simulink model "cantoni_combined_matrices_6pools_split"  (R2019b)
settings: Solver=FixedStepDiscrete  StartTime=0.0  StopTime=30000  FixedStep=h  RelTol=1e-3
undefined symbols (not defined in the file or in its folder): comb_contr, comb_plant_disc, ddelay, h, Pd, Wd
settings Model: Creator=Jacob  LastModifiedBy=bas
settings SFSimCC: CustomCodeUndefinedFunction=UseInterfaceOnly

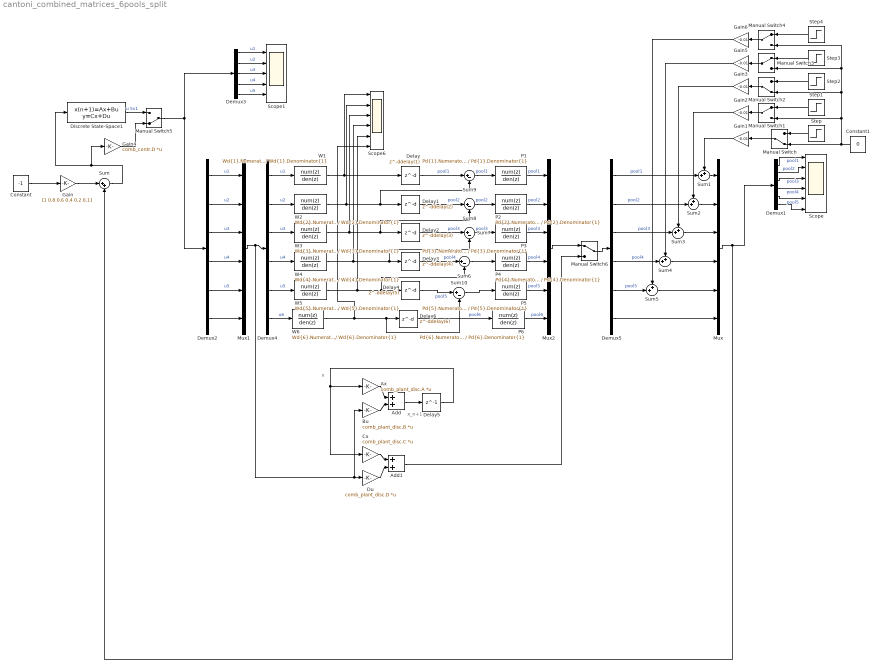
== system cantoni_combined_matrices_6pools_split ==
  note: x
  note: x_n+1
  Add : Sum
  Add1 : Sum
  Ax : Gain  Gain=comb_plant_disc.A  Multiplication=Matrix(K*u)
  Bu : Gain  Gain=comb_plant_disc.B  Multiplication=Matrix(K*u)
  Constant : Constant  Value=-1
  Constant1 : Constant  Value=0
  Cx : Gain  Gain=comb_plant_disc.C  Multiplication=Matrix(K*u)
  Delay : Delay  DelayLength=ddelay(1)
  Delay1 : Delay  DelayLength=ddelay(2)
  Delay2 : Delay  DelayLength=ddelay(3)
  Delay3 : Delay  DelayLength=ddelay(4)
  Delay4 : Delay  DelayLength=ddelay(5)
  Delay5 : Delay  DelayLength=1  InitialCondition=[0;0;0;0;0;0;0;0;0;0;0;0;0;0;0;0;0;0;0;0;0;0;0;0]
  Delay6 : Delay  DelayLength=ddelay(6)
  Demux{1..2,4..5} (4 alike) : Demux  Outputs=6
  Demux3 : Demux  Outputs=5
  Discrete State-Space1 : DiscreteStateSpace  A=comb_contr.A  B=comb_contr.B  C=comb_contr.C  D=comb_contr.D  SampleTime=h
  Du : Gain  Gain=comb_plant_disc.D  Multiplication=Matrix(K*u)
  Gain : Gain  Gain=[1 0.8 0.6 0.4 0.2 0.1]
  Gain{1..3,5..6} (5 alike) : Gain  Gain=-0.01
  Gain4 : Gain  Gain=comb_contr.D  Multiplication=Matrix(K*u)
  Manual Switch : ManualSwitch  CurrentSetting=0
  Manual Switch{1,3..4,6} (4 alike) : ManualSwitch
  Manual Switch2 : ManualSwitch  CurrentSetting=0
  Manual Switch5 : ManualSwitch  CurrentSetting=0
  Mux : Mux  Inputs=6
  Mux1 : Mux  Inputs=6
  Mux2 : Mux  Inputs=6
  P1 : DiscreteTransferFcn  Numerator=Pd{1}.Numerator{1}  Denominator=Pd{1}.Denominator{1}
  P2 : DiscreteTransferFcn  Numerator=Pd{2}.Numerator{1}  Denominator=Pd{2}.Denominator{1}
  P3 : DiscreteTransferFcn  Numerator=Pd{3}.Numerator{1}  Denominator=Pd{3}.Denominator{1}
  P4 : DiscreteTransferFcn  Numerator=Pd{4}.Numerator{1}  Denominator=Pd{4}.Denominator{1}
  P5 : DiscreteTransferFcn  Numerator=Pd{5}.Numerator{1}  Denominator=Pd{5}.Denominator{1}
  P6 : DiscreteTransferFcn  Numerator=Pd{6}.Numerator{1}  Denominator=Pd{6}.Denominator{1}
  Scope : Scope  NumInputPorts=6
  Scope1 : Scope  NumInputPorts=5
  Scope6 : Scope  NumInputPorts=6
  Step{,1..4} (5 alike) : Step  Time=50  SampleTime=0
  Sum : Sum  Inputs=|++
  Sum{1..5} (5 alike) : Sum  Inputs=++|
  Sum{6..10} (5 alike) : Sum  Inputs=|+-
  W1 : DiscreteTransferFcn  Numerator=Wd{1}.Numerator{1}  Denominator=Wd{1}.Denominator{1}
  W2 : DiscreteTransferFcn  Numerator=Wd{2}.Numerator{1}  Denominator=Wd{2}.Denominator{1}
  W3 : DiscreteTransferFcn  Numerator=Wd{3}.Numerator{1}  Denominator=Wd{3}.Denominator{1}
  W4 : DiscreteTransferFcn  Numerator=Wd{4}.Numerator{1}  Denominator=Wd{4}.Denominator{1}
  W5 : DiscreteTransferFcn  Numerator=Wd{5}.Numerator{1}  Denominator=Wd{5}.Denominator{1}
  W6 : DiscreteTransferFcn  Numerator=Wd{6}.Numerator{1}  Denominator=Wd{6}.Denominator{1}
  wires:
  Sum/1 -> Gain4/1, Discrete State-Space1/1
  Constant/1 -> Gain/1
  Gain/1 -> Sum/1
  Mux/1 -> Demux1/1, Sum/2
  Demux1/1 -> Scope/1  "pool1"
  Demux1/2 -> Scope/2  "pool2"
  Demux1/3 -> Scope/3  "pool3"
  Demux1/4 -> Scope/4  "pool4"
  Demux1/5 -> Scope/5  "pool5"
  Step/1 -> Manual Switch/1
  Sum1/1 -> Mux/1
  Demux5/2 -> Sum2/2  "pool2"
  Sum2/1 -> Mux/2
  Gain2/1 -> Sum2/1
  Step1/1 -> Manual Switch1/1
  Gain1/1 -> Sum1/1
  Manual Switch/1 -> Gain1/1
  Constant1/1 -> Manual Switch1/2, Manual Switch4/2, Manual Switch3/2, Manual Switch2/2, Manual Switch/2
  Manual Switch1/1 -> Gain2/1
  Demux5/3 -> Sum3/2  "pool3"
  Sum3/1 -> Mux/3
  Manual Switch2/1 -> Gain3/1
  Step2/1 -> Manual Switch2/1
  Gain3/1 -> Sum3/1
  Demux5/1 -> Sum1/2  "pool1"
  Demux5/4 -> Sum4/2  "pool4"
  Sum4/1 -> Mux/4
  Demux5/5 -> Sum5/2  "pool5"
  Sum5/1 -> Mux/5
  Step3/1 -> Manual Switch3/1
  Manual Switch3/1 -> Gain5/1
  Gain5/1 -> Sum4/1
  Manual Switch4/1 -> Gain6/1
  Step4/1 -> Manual Switch4/1
  Gain6/1 -> Sum5/1
  Demux2/4 -> Mux1/4  "u4"
  Demux2/3 -> Mux1/3  "u3"
  Demux2/2 -> Mux1/2  "u2"
  Demux2/1 -> Mux1/1  "u1"
  Demux2/5 -> Mux1/5  "u5"
  Demux3/5 -> Scope1/5  "u5"
  Demux3/4 -> Scope1/4  "u4"
  Demux3/3 -> Scope1/3  "u3"
  Demux3/2 -> Scope1/2  "u2"
  Demux3/1 -> Scope1/1  "u1"
  W5/1 -> Sum6/2, Delay4/1, Scope6/5
  Discrete State-Space1/1 -> Manual Switch5/1  "u 5x1"
  Manual Switch5/1 -> Demux3/1, Demux2/1
  Gain4/1 -> Manual Switch5/2
  Demux4/1 -> W1/1  "u1"
  Demux4/2 -> W2/1  "u2"
  Demux4/3 -> W3/1  "u3"
  Demux4/4 -> W4/1  "u4"
  Demux4/5 -> W5/1  "u5"
  Mux2/1 -> Manual Switch6/1
  P1/1 -> Mux2/1  "pool1"
  P2/1 -> Mux2/2  "pool2"
  P3/1 -> Mux2/3  "pool3"
  P4/1 -> Mux2/4  "pool4"
  P5/1 -> Mux2/5  "pool5"
  Add1/1 -> Manual Switch6/2
  Manual Switch6/1 -> Demux5/1
  Sum6/1 -> P4/1
  W4/1 -> Sum7/2, Delay3/1, Scope6/4
  W1/1 -> Delay/1, Scope6/1
  W2/1 -> Sum9/2, Delay1/1, Scope6/2
  W3/1 -> Sum8/2, Delay2/1, Scope6/3
  Bu/1 -> Add/2
  Ax/1 -> Add/1
  Delay5/1 -> Cx/1, Ax/1
  Du/1 -> Add1/2
  Add/1 -> Delay5/1
  Cx/1 -> Add1/1
  Mux1/1 -> Du/1, Bu/1, Demux4/1
  Sum9/1 -> P1/1  "pool1"
  Sum8/1 -> P2/1  "pool2"
  Sum7/1 -> P3/1  "pool3"
  Delay/1 -> Sum9/1  "pool1"
  Delay1/1 -> Sum8/1  "pool2"
  Delay2/1 -> Sum7/1  "pool3"
  Delay3/1 -> Sum6/1  "pool4"
  Demux5/6 -> Mux/6
  Demux1/6 -> Scope/6
  Demux2/6 -> Mux1/6
  Delay6/1 -> P6/1  "pool6"
  Demux4/6 -> W6/1  "u6"
  W6/1 -> Scope6/6, Sum10/2, Delay6/1
  P6/1 -> Mux2/6  "pool6"
  Sum10/1 -> P5/1
  Delay4/1 -> Sum10/1  "pool5"
